simulink model "orig_recieve_udp"  (R2014b)
settings: Solver=ode3  StartTime=0.0  StopTime=inf  RelTol=1e-3
libraries: xpcutilitieslib x1, slrtlib x1
settings Model: SimulationMode=external  BufferReuse=off  Creator=Boreth  LastModifiedBy=Boreth
settings SolverCC: EnableConcurrentExecution=on
settings OptimizationCC: BlockReduction=off  OptimizeBlockIOStorage=off  BufferReuse=off  GlobalBufferReuse=off  ExpressionFolding=off  LocalBlockOutputs=off
settings HardwareCC: ProdIntDivRoundTo=Zero  ProdEndianess=LittleEndian  ProdLongLongMode=on  ProdHWDeviceType=Generic->32-bit x86 compatible
settings RTWCC: SystemTargetFile=slrt.tlc  TemplateMakefile=slrt_default_tmf  Description=Simulink Real-Time  ProcessScript=slrt_make_rtw_hook  RTWCompilerOptimization=On
settings SimulinkRealTimeCC: GeneratePreprocessorConditionals=Disable all  EnableShiftOperators=on

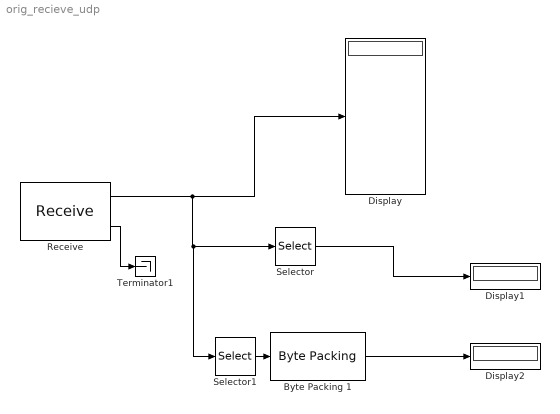
== system orig_recieve_udp ==
  Byte Packing 1 : xpcutilitieslib/Byte Packing   MaskPackedDataType=single  MaskUnpackedDataTypes={'uint8'}  MaskAlignment=4
  Display : Display
  Display1 : Display
  Display2 : Display
  "Receive " : slrtlib/UDP/Receive   ipAddress=192.168.1.100  ipPort=50002  width=5  vblLen=on  sampletime=0.1
  Selector : Selector  InputPortWidth=5
  Selector1 : Selector  InputPortWidth=5  Indices=[2:5]
  Terminator1 : Terminator
  wires:
  "Receive "/2 -> Terminator1/1
  "Receive "/1 -> Selector1/1, Selector/1, Display/1
  Byte Packing 1/1 -> Display2/1
  Selector/1 -> Display1/1
  Selector1/1 -> Byte Packing 1/1
